simulink model "SuperState"  (R2018b)
settings: Solver=FixedStepDiscrete  StartTime=0.0  StopTime=10.0  FixedStep=0.01  RelTol=1e-3
settings Model: Creator=marwan  LastModifiedBy=marwan

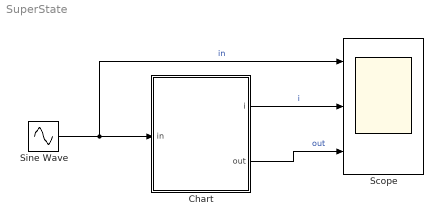
== system SuperState ==
  Chart : Stateflow chart  TreatAsAtomicUnit=on
  Scope : Scope  NumInputPorts=3
  Sine Wave : Sin  Amplitude=2  SampleTime=0
  wires:
  Sine Wave/1 -> Scope/1, Chart/1(in)  "in"
  Chart/1(i) -> Scope/2  "i"
  Chart/2(out) -> Scope/3  "out"

== stateflow chart SuperState/Chart ==
  state off
    en: out=0;
    state def
      en: i=0;
    state before_switch_
      during: i=i+1;
    (default) -> off.def
    off.before_switch_ -> off.def : [in<0]
    off.def -> off.before_switch_ : [in>0]
  state on
    en: out=1;
    state def
      en: i=0;
    state before_switch_
      during: i=i+1;
    (default) -> on.def
    on.before_switch_ -> on.def : [in>0]
    on.def -> on.before_switch_ : [in<0]
  note: subchart
  (default) -> off
  off -> on.def : [i>=40]
  on -> off.def : [i>=40]
  data: in input; i output; out output
